simulink model "gm_uz_pmsm_model_6LUT_pd_vnl"  (R2023b)
settings: Solver=FixedStepAuto  StartTime=0.0  StopTime=0.05  RelTol=1e-3
PreLoadFcn:
  | uz_pmsm_model_init_parameter
PostLoadFcn:
  | % Import the data from Excel for a lookup table
  | FluxMapData = readtable('C:\Users\Philipp\ultrazohm\ultrazohm_sw\ip_cores\uz_pmsm_model\FluxMapData_2023-05-26_13-07-57.csv');
  | % Row indices for lookup table
  | d_current_in_d_axis = FluxMapData(8:27,1:end);
  | % Column indices for lookup table
  | q_current_in_d_axis = FluxMapData(29:48,1:end);
  | % Output values for lookup table
  | d_Flux_d_axis = FluxMapData(50:69,1:end);
undefined symbols (not defined in the file or in its folder): ad1, ad2, ad3, ad4, ad5, ad6, aq1, aq2, aq3, aq4, aq5, aq6, d_current_d_Flux, d_current_q_Flux, entkopplung_dynamic, entkopplung_linear, entkopplung_static, Fid1_Giq1, Fid2_Giq2, Flux_d, Flux_q, friction_coefficient, inertia, Ki_Bo_d, Ki_Bo_q, Kp_Bo_d, Kp_Bo_q, L_d, L_q, Ldq, parameter_nachfuerung, polepair, praediktion_entkopplung_nonlinear, psi_pm, q_current_d_Flux, q_current_q_Flux, R_1, simulate_mechanical, simulate_nonlinear_modell, simulate_open_loop, static_friction_torque, tau_sum, ts, ts_regler
libraries: hdlmdlgenlib x19, simulink x2, slpidlib x2
(part 2 of 4)

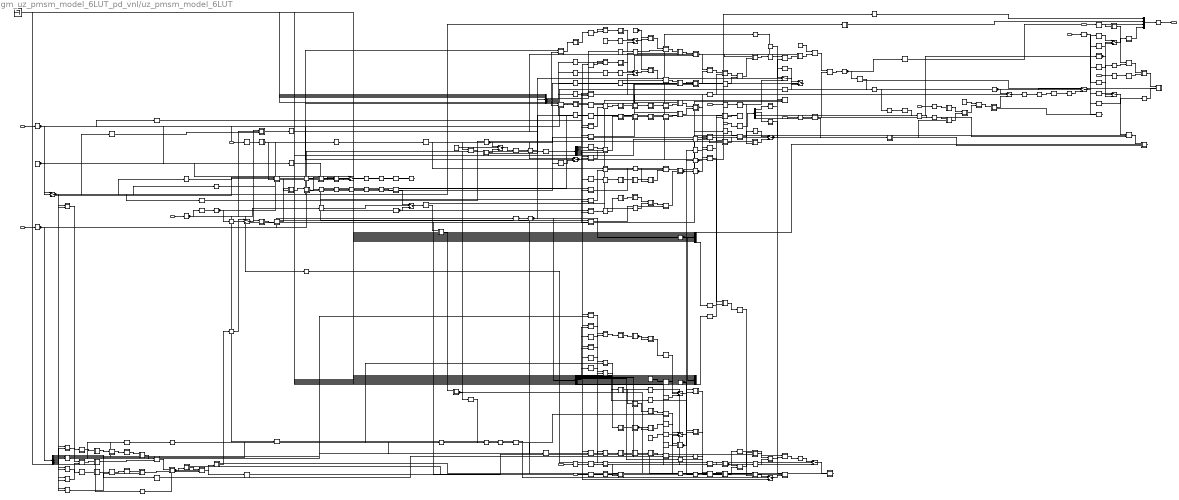
== system gm_uz_pmsm_model_6LUT_pd_vnl/uz_pmsm_model_6LUT ==
  reset_integrators : Inport  OutDataTypeStr=boolean  PortDimensions=1  SampleTime=2e-06
  simulate_mechanical : Inport  Port=2  OutDataTypeStr=boolean  PortDimensions=1  SampleTime=2e-06
  simulate_nonlinear : Inport  Port=3  OutDataTypeStr=boolean  PortDimensions=1  SampleTime=2e-06
  reciprocal_J : Inport  Port=4  OutDataTypeStr=single  PortDimensions=1  SampleTime=2e-06
  mu : Inport  Port=5  OutDataTypeStr=single  PortDimensions=1  SampleTime=2e-06
  M_n0 : Inport  Port=6  OutDataTypeStr=single  PortDimensions=1  SampleTime=2e-06
  R1 : Inport  Port=7  OutDataTypeStr=single  PortDimensions=1  SampleTime=2e-06
  polepairs : Inport  Port=8  OutDataTypeStr=single  PortDimensions=1  SampleTime=2e-06
  Ld : Inport  Port=9  OutDataTypeStr=single  PortDimensions=1  SampleTime=2e-06
  Lq : Inport  Port=10  OutDataTypeStr=single  PortDimensions=1  SampleTime=2e-06
  psi_pm : Inport  Port=11  OutDataTypeStr=single  PortDimensions=1  SampleTime=2e-06
  fitting_parameters : Inport  Port=12  OutDataTypeStr=double  PortDimensions=[14]  SampleTime=2e-06
  inputs : Inport  Port=13  OutDataTypeStr=single  PortDimensions=[4]  SampleTime=2e-06
  Abs : Subsystem
      mask Display: disp('NFP\nabs');
  Constant : Constant  Value=double(0)  OutDataTypeStr=double  SampleTime=1e-08
  Constant1 : Constant  Value=double(1)  OutDataTypeStr=double  SampleTime=1e-08
  Constant11 : Constant  Value=double(1)  OutDataTypeStr=double  SampleTime=1e-08
  Data Type Conversion1 : Subsystem
      mask Display: disp('NFP\nconv');
  Data Type Conversion10 : Subsystem
      mask Display: disp('NFP\nconv');
  Data Type Conversion11 : Subsystem
      mask Display: disp('NFP\nconv');
  Data Type Conversion111 : Subsystem
      mask Display: disp('NFP\nconv');
  Data Type Conversion12 : Subsystem
      mask Display: disp('NFP\nconv');
  Data Type Conversion121 : Subsystem
      mask Display: disp('NFP\nconv');
  Data Type Conversion13 : Subsystem
      mask Display: disp('NFP\nconv');
  Data Type Conversion14 : Subsystem
      mask Display: disp('NFP\nconv');
  Data Type Conversion15 : Subsystem
      mask Display: disp('NFP\nconv');
  Data Type Conversion16 : Subsystem
      mask Display: disp('NFP\nconv');
  Data Type Conversion17 : Subsystem
      mask Display: disp('NFP\nconv');
  Data Type Conversion2 : Subsystem
      mask Display: disp('NFP\nconv');
  Data Type Conversion21 : Subsystem
      mask Display: disp('NFP\nconv');
  Data Type Conversion22 : Subsystem
      mask Display: disp('NFP\nconv');
  Data Type Conversion23 : Subsystem
      mask Display: disp('NFP\nconv');
  Data Type Conversion24 : Subsystem
      mask Display: disp('NFP\nconv');
  Data Type Conversion3 : Subsystem
      mask Display: disp('NFP\nconv');
  Data Type Conversion31 : Subsystem
      mask Display: disp('NFP\nconv');
  Data Type Conversion32 : Subsystem
      mask Display: disp('NFP\nconv');
  Data Type Conversion4 : Subsystem
      mask Display: disp('NFP\nconv');
  Data Type Conversion41 : Subsystem
      mask Display: disp('NFP\nconv');
  Data Type Conversion42 : Subsystem
      mask Display: disp('NFP\nconv');
  Data Type Conversion43 : Subsystem
      mask Display: disp('NFP\nconv');
  Data Type Conversion5 : Subsystem
      mask Display: disp('NFP\nconv');
  Data Type Conversion51 : Subsystem
      mask Display: disp('NFP\nconv');
  Data Type Conversion52 : Subsystem
      mask Display: disp('NFP\nconv');
  Data Type Conversion53 : Subsystem
      mask Display: disp('NFP\nconv');
  Data Type Conversion6 : Subsystem
      mask Display: disp('NFP\nconv');
  Data Type Conversion61 : Subsystem
      mask Display: disp('NFP\nconv');
  Data Type Conversion62 : Subsystem
      mask Display: disp('NFP\nconv');
  Data Type Conversion63 : Subsystem
      mask Display: disp('NFP\nconv');
  Data Type Conversion64 : Subsystem
      mask Display: disp('NFP\nconv');
  Data Type Conversion7 : Subsystem
      mask Display: disp('NFP\nconv');
  Data Type Conversion71 : Subsystem
      mask Display: disp('NFP\nconv');
  Data Type Conversion72 : Subsystem
      mask Display: disp('NFP\nconv');
  Data Type Conversion8 : Subsystem
      mask Display: disp('NFP\nconv');
  Data Type Conversion81 : Subsystem
      mask Display: disp('NFP\nconv');
  Data Type Conversion82 : Subsystem
      mask Display: disp('NFP\nconv');
  Data Type Conversion83 : Subsystem
      mask Display: disp('NFP\nconv');
  Data Type Conversion9 : Subsystem
      mask Display: disp('NFP\nconv');
  Delay : RateTransition  OutPortSampleTimeOpt=Multiple of input port sample time  OutPortSampleTimeMultiple=200
  Delay1_lowered : RateTransition  OutPortSampleTimeOpt=Multiple of input port sample time  OutPortSampleTimeMultiple=200
  Delay1_lowered1 : RateTransition  OutPortSampleTimeOpt=Multiple of input port sample time  OutPortSampleTimeMultiple=200
  Delay1_lowered2 : RateTransition  OutPortSampleTimeOpt=Multiple of input port sample time  OutPortSampleTimeMultiple=200
  Delay1_lowered_absorbed : Delay  DelayLength=0
  Delay1_lowered_absorbed1 : Delay  DelayLength=0
  Delay1_lowered_absorbed2 : Delay  DelayLength=0
  Delay_absorbed : Delay  DelayLength=0
  Divide : Subsystem
      mask Display: disp('NFP\nmul');
  Divide1 : Subsystem
      mask Display: disp('NFP\nmul');
  Divide_recip : Subsystem
      mask Display: disp('NFP\nmath');
  Factor : Subsystem
      mask Display: disp('NFP\nmul');
  Factor_const : Constant  Value=double(1.5)  OutDataTypeStr=double  SampleTime=1e-08
  From1 : hdlmdlgenlib/Buffer
  From1_out1_0_term0 : Terminator
  From1_out1_10_term10 : Terminator
  From1_out1_11_term11 : Terminator
  From1_out1_12_term12 : Terminator
  From1_out1_13_term13 : Terminator
  From1_out1_1_term1 : Terminator
  From1_out1_2_term2 : Terminator
  From1_out1_3_term3 : Terminator
  From1_out1_4_term4 : Terminator
  From1_out1_5_term5 : Terminator
  From1_out1_6_term6 : Terminator
  From1_out1_7_term7 : Terminator
  From1_out1_8_term8 : Terminator
  From1_out1_9_term9 : Terminator
  From2 : hdlmdlgenlib/Buffer
  From2_out1_0_term0 : Terminator
  From2_out1_0_term01 : Terminator
  From2_out1_10_term10 : Terminator
  From2_out1_10_term101 : Terminator
  From2_out1_11_term11 : Terminator
  From2_out1_11_term111 : Terminator
  From2_out1_12_term12 : Terminator
  From2_out1_13_term13 : Terminator
  From2_out1_1_term1 : Terminator
  From2_out1_1_term11 : Terminator
  From2_out1_2_term2 : Terminator
  From2_out1_2_term21 : Terminator
  From2_out1_3_term3 : Terminator
  From2_out1_3_term31 : Terminator
  From2_out1_4_term4 : Terminator
  From2_out1_4_term41 : Terminator
  From2_out1_5_term5 : Terminator
  From2_out1_5_term51 : Terminator
  From2_out1_6_term6 : Terminator
  From2_out1_6_term61 : Terminator
  From2_out1_7_term7 : Terminator
  From2_out1_7_term71 : Terminator
  From2_out1_8_term8 : Terminator
  From2_out1_8_term81 : Terminator
  From2_out1_9_term9 : Terminator
  From2_out1_9_term91 : Terminator
  From3 : hdlmdlgenlib/Buffer
  Gain : Subsystem
      mask Display: disp('NFP\nmul');
  Gain7 : Subsystem
      mask Display: disp('NFP\nmul');
  Gain71 : Subsystem
      mask Display: disp('NFP\nmul');
  Gain7_const : Constant  Value=double(2e-06)  OutDataTypeStr=double  SampleTime=1e-08
  Gain7_const1 : Constant  Value=double(2e-06)  OutDataTypeStr=double  SampleTime=1e-08
  Gain_const : Constant  Value=double(2e-06)  OutDataTypeStr=double  SampleTime=1e-08
  Gain_unaryminus : Subsystem
      mask Display: disp('NFP\numinus');
  Gain_unaryminus1 : Subsystem
      mask Display: disp('NFP\numinus');
  Goto1 : hdlmdlgenlib/Buffer
  Goto2 : hdlmdlgenlib/Buffer
  Initial_Val : Constant  Value=double(0)  OutDataTypeStr=double  SampleTime=1e-08
  Initial_Val1 : Constant  Value=double(0)  OutDataTypeStr=double  SampleTime=1e-08
  Initial_Val2 : Constant  Value=double(0)  OutDataTypeStr=double  SampleTime=1e-08
  Ldd : hdlmdlgenlib/Buffer
  Log : Subsystem
      mask Display: disp('NFP\nmath');
  Log1 : Subsystem
      mask Display: disp('NFP\nmath');
  Log11 : Subsystem
      mask Display: disp('NFP\nmath');
  Log2 : Subsystem
      mask Display: disp('NFP\nmath');
  Lqq : hdlmdlgenlib/Buffer
  M_Mi : hdlmdlgenlib/Buffer
  Product : Subsystem
      mask Display: disp('NFP\nmul');
  Product1 : Subsystem
      mask Display: disp('NFP\nmul');
  Product10 : Subsystem
      mask Display: disp('NFP\nmul');
  Product101 : Subsystem
      mask Display: disp('NFP\nmul');
  Product102 : Subsystem
      mask Display: disp('NFP\nmul');
  Product103 : Subsystem
      mask Display: disp('NFP\nmul');
  Product104 : Subsystem
      mask Display: disp('NFP\nmul');
  Product105 : Subsystem
      mask Display: disp('NFP\nmul');
  Product11 : Subsystem
      mask Display: disp('NFP\nmul');
  Product110 : Subsystem
      mask Display: disp('NFP\nmul');
  Product111 : Subsystem
      mask Display: disp('NFP\nmul');
  Product112 : Subsystem
      mask Display: disp('NFP\nmul');
  Product113 : Subsystem
      mask Display: disp('NFP\nmul');
  Product12 : Subsystem
      mask Display: disp('NFP\nmul');
  Product121 : Subsystem
      mask Display: disp('NFP\nmul');
  Product122 : Subsystem
      mask Display: disp('NFP\nmul');
  Product13 : Subsystem
      mask Display: disp('NFP\nmul');
  Product131 : Subsystem
      mask Display: disp('NFP\nmul');
  Product132 : Subsystem
      mask Display: disp('NFP\nmul');
  Product133 : Subsystem
      mask Display: disp('NFP\nmul');
  Product14 : Subsystem
      mask Display: disp('NFP\nmul');
  Product141 : Subsystem
      mask Display: disp('NFP\nmul');
  Product15 : Subsystem
      mask Display: disp('NFP\nmul');
  Product151 : Subsystem
      mask Display: disp('NFP\nmul');
  Product16 : Subsystem
      mask Display: disp('NFP\nmul');
  Product161 : Subsystem
      mask Display: disp('NFP\nmul');
  Product162 : Subsystem
      mask Display: disp('NFP\nmul');
  Product17 : Subsystem
      mask Display: disp('NFP\nmul');
  Product18 : Subsystem
      mask Display: disp('NFP\nmul');
  Product19 : Subsystem
      mask Display: disp('NFP\nmul');
  Product2 : Subsystem
      mask Display: disp('NFP\nmul');
  Product20 : Subsystem
      mask Display: disp('NFP\nmul');
  Product201 : Subsystem
      mask Display: disp('NFP\nmul');
  Product202 : Subsystem
      mask Display: disp('NFP\nmul');
  Product203 : Subsystem
      mask Display: disp('NFP\nmul');
  Product204 : Subsystem
      mask Display: disp('NFP\nmul');
  Product205 : Subsystem
      mask Display: disp('NFP\nmul');
  Product206 : Subsystem
      mask Display: disp('NFP\nmul');
  Product207 : Subsystem
      mask Display: disp('NFP\nmul');
  Product21 : Subsystem
      mask Display: disp('NFP\nmul');
  Product211 : Subsystem
      mask Display: disp('NFP\nmul');
  Product22 : Subsystem
      mask Display: disp('NFP\nmul');
  Product23 : Subsystem
      mask Display: disp('NFP\nmul');
  Product24 : Subsystem
      mask Display: disp('NFP\nmul');
  Product25 : Subsystem
      mask Display: disp('NFP\nmul');
  Product3 : Subsystem
      mask Display: disp('NFP\nmul');
  Product31 : Subsystem
      mask Display: disp('NFP\nmul');
  Product32 : Subsystem
      mask Display: disp('NFP\nmul');
  Product33 : Subsystem
      mask Display: disp('NFP\nmul');
  Product34 : Subsystem
      mask Display: disp('NFP\nmul');
  Product35 : Subsystem
      mask Display: disp('NFP\nmul');
  Product36 : Subsystem
      mask Display: disp('NFP\nmul');
  Product37 : Subsystem
      mask Display: disp('NFP\nmul');
  Product4 : Subsystem
      mask Display: disp('NFP\nmul');
  Product41 : Subsystem
      mask Display: disp('NFP\nmul');
  Product42 : Subsystem
      mask Display: disp('NFP\nmul');
  Product43 : Subsystem
      mask Display: disp('NFP\nmul');
  Product5 : Subsystem
      mask Display: disp('NFP\nmul');
  Product51 : Subsystem
      mask Display: disp('NFP\nmul');
  Product52 : Subsystem
      mask Display: disp('NFP\nmul');
  Product6 : Subsystem
      mask Display: disp('NFP\nmul');
  Product61 : Subsystem
      mask Display: disp('NFP\nmul');
  Product7 : Subsystem
      mask Display: disp('NFP\nmul');
  Product71 : Subsystem
      mask Display: disp('NFP\nmul');
  Product7_to_gain : Subsystem
      mask Display: disp('NFP\ngain_pow2');
  Product8 : Subsystem
      mask Display: disp('NFP\nmul');
  Product81 : Subsystem
      mask Display: disp('NFP\nmul');
  Product9 : Subsystem
      mask Display: disp('NFP\nmul');
  Product91 : Subsystem
      mask Display: disp('NFP\nmul');
  Product92 : Subsystem
      mask Display: disp('NFP\nmul');
  Product93 : Subsystem
      mask Display: disp('NFP\nmul');
  Product94 : Subsystem
      mask Display: disp('NFP\nmul');
  Sign1 : Subsystem
      mask Display: disp('NFP\nsignum');
  Sum : Subsystem
      mask Display: disp('NFP\nadd');
  Sum1 : Subsystem
      mask Display: disp('NFP\nadd');
  Sum10 : Subsystem
      mask Display: disp('NFP\nadd');
  Sum101 : Subsystem
      mask Display: disp('NFP\nadd');
  Sum11 : Subsystem
      mask Display: disp('NFP\nadd');
  Sum12 : Subsystem
      mask Display: disp('NFP\nadd');
  Sum13 : Subsystem
      mask Display: disp('NFP\nadd');
  Sum14 : Subsystem
      mask Display: disp('NFP\nadd');
  Sum2 : Subsystem
      mask Display: disp('NFP\nadd');
  Sum21 : Subsystem
      mask Display: disp('NFP\nadd');
  Sum22 : Subsystem
      mask Display: disp('NFP\nadd');
  Sum23 : Subsystem
      mask Display: disp('NFP\nadd');
  Sum24 : Subsystem
      mask Display: disp('NFP\nadd');
  Sum3 : Subsystem
      mask Display: disp('NFP\nadd');
  Sum31 : Subsystem
      mask Display: disp('NFP\nadd');
  Sum32 : Subsystem
      mask Display: disp('NFP\nadd');
  Sum3_stage2 : Subsystem
      mask Display: disp('NFP\nadd');
  Sum3_stage21 : Subsystem
      mask Display: disp('NFP\nadd');
  Sum3_stage3 : Subsystem
      mask Display: disp('NFP\nadd');
  Sum3_stage31 : Subsystem
      mask Display: disp('NFP\nadd');
  Sum3_stage4 : Subsystem
      mask Display: disp('NFP\nadd');
  Sum4 : Subsystem
      mask Display: disp('NFP\nadd');
  Sum41 : Subsystem
      mask Display: disp('NFP\nadd');
  Sum42 : Subsystem
      mask Display: disp('NFP\nadd');
  Sum4_stage2 : Subsystem
      mask Display: disp('NFP\nadd');
  Sum4_stage3 : Subsystem
      mask Display: disp('NFP\nadd');
  Sum4_stage4 : Subsystem
      mask Display: disp('NFP\nadd');
  Sum5 : Subsystem
      mask Display: disp('NFP\nadd');
  Sum51 : Subsystem
      mask Display: disp('NFP\nadd');
  Sum52 : Subsystem
      mask Display: disp('NFP\nadd');
  Sum53 : Subsystem
      mask Display: disp('NFP\nadd');
  Sum6 : Subsystem
      mask Display: disp('NFP\nadd');
  Sum7 : Subsystem
      mask Display: disp('NFP\nadd');
  Sum71 : Subsystem
      mask Display: disp('NFP\nadd');
  Sum8 : Subsystem
      mask Display: disp('NFP\nadd');
  Sum9 : Subsystem
      mask Display: disp('NFP\nadd');
  Switch{,1..6,11} (8 alike) : Switch  Criteria=u2 ~= 0  Threshold=double(0)  OutDataTypeStr=double  SampleTime=1e-08  SaturateOnIntegerOverflow=off  InputSameDT=off
  Tanh : Subsystem
      mask Display: disp('NFP\ntrig');
  Tanh1 : Subsystem
      mask Display: disp('NFP\ntrig');
  Tanh11 : Subsystem
      mask Display: disp('NFP\ntrig');
  Tanh12 : Subsystem
      mask Display: disp('NFP\ntrig');
  Tanh13 : Subsystem
      mask Display: disp('NFP\ntrig');
  Tanh2 : Subsystem
      mask Display: disp('NFP\ntrig');
  Tanh21 : Subsystem
      mask Display: disp('NFP\ntrig');
  Tanh3 : Subsystem
      mask Display: disp('NFP\ntrig');
  Tanh31 : Subsystem
      mask Display: disp('NFP\ntrig');
  Tanh4 : Subsystem
      mask Display: disp('NFP\ntrig');
  Tanh41 : Subsystem
      mask Display: disp('NFP\ntrig');
  Tanh5 : Subsystem
      mask Display: disp('NFP\ntrig');
  Unit Delay : RateTransition  OutPortSampleTimeOpt=Multiple of input port sample time  OutPortSampleTimeMultiple=200
  Unit Delay1 : RateTransition  OutPortSampleTimeOpt=Multiple of input port sample time  OutPortSampleTimeMultiple=200
  Unit Delay1_absorbed : Delay  DelayLength=0
  Unit Delay_absorbed : Delay  DelayLength=0
  crp_out_delay{,1..5} (6 alike) : Delay  DelayLength=double(1)  InitialCondition=0  SampleTime=1e-08
  default_value{,1..4} (5 alike) : Constant  Value=double(1)  OutDataTypeStr=double  SampleTime=1e-08
  delayMatch{,1..16,18..20,22..41,43..45,47..51,53..57} (53 alike) : Delay  DelayLength=double(1)  InitialCondition=0  SampleTime=1e-08
  delayMatch17 : Delay  DelayLength=double(41)  InitialCondition=0  SampleTime=1e-08
  delayMatch21 : Delay  DelayLength=double(41)  InitialCondition=0  SampleTime=1e-08
  delayMatch42 : Delay  DelayLength=double(35)  InitialCondition=0  SampleTime=1e-08
  delayMatch46 : Delay  DelayLength=double(35)  InitialCondition=0  SampleTime=1e-08
  delayMatch52 : Delay  DelayLength=double(108)  InitialCondition=0  SampleTime=1e-08
  fitting_parameters_12_term12 : Terminator
  fitting_parameters_13_term13 : Terminator
  in0_repeat : RateTransition  Integrity=off  Deterministic=off  OutPortSampleTimeOpt=Multiple of input port sample time  OutPortSampleTimeMultiple=1/200
  in10_repeat : RateTransition  Integrity=off  Deterministic=off  OutPortSampleTimeOpt=Multiple of input port sample time  OutPortSampleTimeMultiple=1/200
  in11_repeat : RateTransition  Integrity=off  Deterministic=off  OutPortSampleTimeOpt=Multiple of input port sample time  OutPortSampleTimeMultiple=1/200
  in12_repeat : RateTransition  Integrity=off  Deterministic=off  OutPortSampleTimeOpt=Multiple of input port sample time  OutPortSampleTimeMultiple=1/200
  in13_repeat : RateTransition  Integrity=off  Deterministic=off  OutPortSampleTimeOpt=Multiple of input port sample time  OutPortSampleTimeMultiple=1/200
  in14_repeat : RateTransition  Integrity=off  Deterministic=off  OutPortSampleTimeOpt=Multiple of input port sample time  OutPortSampleTimeMultiple=1/200
  in15_repeat : RateTransition  Integrity=off  Deterministic=off  OutPortSampleTimeOpt=Multiple of input port sample time  OutPortSampleTimeMultiple=1/200
  in16_repeat : RateTransition  Integrity=off  Deterministic=off  OutPortSampleTimeOpt=Multiple of input port sample time  OutPortSampleTimeMultiple=1/200
  in17_repeat : RateTransition  Integrity=off  Deterministic=off  OutPortSampleTimeOpt=Multiple of input port sample time  OutPortSampleTimeMultiple=1/200
  in18_repeat : RateTransition  Integrity=off  Deterministic=off  OutPortSampleTimeOpt=Multiple of input port sample time  OutPortSampleTimeMultiple=1/200
  in1_repeat : RateTransition  Integrity=off  Deterministic=off  OutPortSampleTimeOpt=Multiple of input port sample time  OutPortSampleTimeMultiple=1/200
  in2_repeat : RateTransition  Integrity=off  Deterministic=off  OutPortSampleTimeOpt=Multiple of input port sample time  OutPortSampleTimeMultiple=1/200
  in3_repeat : RateTransition  Integrity=off  Deterministic=off  OutPortSampleTimeOpt=Multiple of input port sample time  OutPortSampleTimeMultiple=1/200
  in4_repeat : RateTransition  Integrity=off  Deterministic=off  OutPortSampleTimeOpt=Multiple of input port sample time  OutPortSampleTimeMultiple=1/200
  in5_repeat : RateTransition  Integrity=off  Deterministic=off  OutPortSampleTimeOpt=Multiple of input port sample time  OutPortSampleTimeMultiple=1/200
  in6_repeat : RateTransition  Integrity=off  Deterministic=off  OutPortSampleTimeOpt=Multiple of input port sample time  OutPortSampleTimeMultiple=1/200
  in7_repeat : RateTransition  Integrity=off  Deterministic=off  OutPortSampleTimeOpt=Multiple of input port sample time  OutPortSampleTimeMultiple=1/200
  in8_repeat : RateTransition  Integrity=off  Deterministic=off  OutPortSampleTimeOpt=Multiple of input port sample time  OutPortSampleTimeMultiple=1/200
  in9_repeat : RateTransition  Integrity=off  Deterministic=off  OutPortSampleTimeOpt=Multiple of input port sample time  OutPortSampleTimeMultiple=1/200
  mux : Mux
  psi_d_approx : hdlmdlgenlib/Buffer
  psi_q_approx : hdlmdlgenlib/Buffer
  reset_in : Switch  Criteria=u2 ~= 0  Threshold=double(0)  OutDataTypeStr=double  SampleTime=1e-08  SaturateOnIntegerOverflow=off  InputSameDT=off
  reset_in1 : Switch  Criteria=u2 ~= 0  Threshold=double(0)  OutDataTypeStr=double  SampleTime=1e-08  SaturateOnIntegerOverflow=off  InputSameDT=off
  reset_in2 : Switch  Criteria=u2 ~= 0  Threshold=double(0)  OutDataTypeStr=double  SampleTime=1e-08  SaturateOnIntegerOverflow=off  InputSameDT=off
  reset_out : Switch  Criteria=u2 ~= 0  Threshold=double(0)  OutDataTypeStr=double  SampleTime=1e-08  SaturateOnIntegerOverflow=off  InputSameDT=off
  reset_out1 : Switch  Criteria=u2 ~= 0  Threshold=double(0)  OutDataTypeStr=double  SampleTime=1e-08  SaturateOnIntegerOverflow=off  InputSameDT=off
  reset_out2 : Switch  Criteria=u2 ~= 0  Threshold=double(0)  OutDataTypeStr=double  SampleTime=1e-08  SaturateOnIntegerOverflow=off  InputSameDT=off
  select_signal{,1..4} (5 alike) : Constant  Value=double(1)  OutDataTypeStr=boolean  SampleTime=1e-08
  t : RateTransition  OutPortSampleTimeOpt=Multiple of input port sample time  OutPortSampleTimeMultiple=200
  t{1..6} (6 alike) : Demux  Outputs=14
  t{8..16} (9 alike) : hdlmdlgenlib/Buffer
  t7 : Demux
  zero_protection{,1..4} (5 alike) : Switch  Criteria=u2 ~= 0  Threshold=double(0)  OutDataTypeStr=double  SampleTime=1e-08  SaturateOnIntegerOverflow=off  InputSameDT=off
  outputs : Outport  SampleTime=2e-06
  wires:
  default_value4/1 -> zero_protection4/3
  zero_protection4/1 -> Divide1/2(In2)
  default_value3/1 -> zero_protection3/3
  zero_protection3/1 -> Product162/2(In2)
  default_value2/1 -> zero_protection2/3
  zero_protection2/1 -> Product133/2(In2)
  default_value1/1 -> zero_protection1/3
  zero_protection1/1 -> Product132/2(In2)
  default_value/1 -> zero_protection/3
  zero_protection/1 -> Product161/2(In2)
  reset_out1/1 -> delayMatch9/1, delayMatch34/1, Sign1/1(In1), Abs/1(In1), delayMatch56/1
  delayMatch57/1 -> reset_in1/2
  reset_out/1 -> Data Type Conversion15/1(In1), delayMatch32/1, Product8/1(In1), Product8/2(In2), Product5/1(In1), Product4/1(In1), Product10/1(In1), Product24/1(In1), Product11/1(In1), Product51/1(In1), Product61/1(In1), Product25/1(In1), delayMatch14/1, delayMatch41/1, delayMatch53/1
  select_signal4/1 -> delayMatch52/1
  select_signal3/1 -> delayMatch46/1
  select_signal2/1 -> delayMatch42/1
  delayMatch51/1 -> Switch11/2
  From3/1 -> delayMatch15/1, delayMatch31/1
  delayMatch54/1 -> reset_in/2
  reset_out2/1 -> Data Type Conversion111/1(In1), delayMatch33/1, Sum/1(In1), Sum1/1(In1), Sum11/1(In1), Sum2/1(In1), Sum3/1(In1), Sum6/1(In1), delayMatch/1, delayMatch30/1, delayMatch27/1
  delayMatch40/1 -> Switch4/2
  delayMatch26/1 -> Switch2/2
  select_signal/1 -> delayMatch21/1
  delayMatch23/1 -> Product32/2(In2)
  select_signal1/1 -> delayMatch17/1
  delayMatch19/1 -> Product19/2(In2)
  delayMatch31/1 -> Switch5/2
  delayMatch41/1 -> Product92/1(In1)
  delayMatch35/1 -> Switch1/2
  delayMatch34/1 -> Switch1/1
  delayMatch30/1 -> Product52/1(In1)
  delayMatch52/1 -> zero_protection4/2
  delayMatch46/1 -> zero_protection3/2
  delayMatch42/1 -> zero_protection2/2
  delayMatch17/1 -> zero_protection1/2
  delayMatch21/1 -> zero_protection/2
  Gain/1(Out1) -> Sum31/1(In1)
  Product7_to_gain/1(Out1) -> Sum3_stage2/2(In2)
  Data Type Conversion14/1(Out1) -> Product93/2(In2), Product131/2(In2)
  Product131/1(Out1) -> Product37/1(In1), Product21/2(In2)
  Sum3_stage4/1(Out1) -> Divide/1(In1)
  Sum3_stage31/1(Out1) -> Sum3_stage4/1(In1)
  Sum3_stage21/1(Out1) -> Sum3_stage31/1(In1)
  Divide_recip/1(Out1) -> Divide/2(In2)
  Sum53/1(Out1) -> reset_in2/3
  Data Type Conversion111/1(Out1) -> mux/1
  Product36/1(Out1) -> Sum32/1(In1)
  Sum32/1(Out1) -> Factor/2(In2)
  Sum9/1(Out1) -> crp_out_delay2/1
  Product43/1(Out1) -> Sum9/2(In2)
  Sum52/1(Out1) -> Product43/1(In1)
  Data Type Conversion64/1(Out1) -> Sum52/2(In2)
  Product122/1(Out1) -> Sum52/1(In1)
  Abs/1(Out1) -> delayMatch36/1
  Sign1/1(Out1) -> delayMatch37/1
  Data Type Conversion121/1(Out1) -> Switch1/3, Switch/3
  Data Type Conversion13/1(Out1) -> Sum14/2(In2)
  Sum14/1(Out1) -> Product112/2(In2)
  Product112/1(Out1) -> Gain/2(In2)
  Data Type Conversion72/1(Out1) -> Product112/1(In1)
  Sum31/1(Out1) -> reset_in1/3
  Data Type Conversion10/1(Out1) -> Sum4_stage2/1(In1)
  Sum4_stage4/1(Out1) -> Divide1/1(In1)
  Sum4_stage3/1(Out1) -> Sum4_stage4/1(In1)
  Sum4_stage2/1(Out1) -> Sum4_stage3/1(In1)
  Sum51/1(Out1) -> reset_in/3
  Product92/1(Out1) -> Sum4_stage4/2(In2)
  Data Type Conversion9/1(Out1) -> Product42/1(In1), Product92/2(In2)
  Product42/1(Out1) -> Sum3_stage21/2(In2)
  Product110/1(Out1) -> Switch6/3
  Sum42/1(Out1) -> Sum24/1(In1), t16/1
  Sum24/1(Out1) -> t11/1, t15/1
  Product206/1(Out1) -> Product207/1(In1)
  Product121/1(Out1) -> Switch3/1
  Product111/1(Out1) -> Switch4/1
  Product204/1(Out1) -> Product205/1(In1)
  Sum23/1(Out1) -> t10/1, t14/1
  Product104/1(Out1) -> Product105/1(In1)
  Sum8/1(Out1) -> Switch5/3
  Data Type Conversion43/1(Out1) -> Sum8/2(In2)
  Product52/1(Out1) -> Sum8/1(In1)
  Data Type Conversion24/1(Out1) -> Switch2/3, Product52/2(In2)
  Product19/1(Out1) -> Sum22/1(In1), t13/1
  Product18/1(Out1) -> Product19/1(In1)
  Product102/1(Out1) -> Product103/1(In1)
  Product16/1(Out1) -> Product17/1(In1)
  Sum13/1(Out1) -> Sum10/1(In1), Sum21/1(In1)
  Product202/1(Out1) -> Product203/1(In1)
  Product20/1(Out1) -> Product201/1(In1)
  Data Type Conversion23/1(Out1) -> Product35/1(In1)
  Tanh13/1(Out1) -> Data Type Conversion23/1(In1)
  Data Type Conversion71/1(Out1) -> Tanh13/1(In1)
  Product25/1(Out1) -> Data Type Conversion71/1(In1)
  Sum12/1(Out1) -> Sum24/2(In2)
  Product61/1(Out1) -> Sum12/2(In2)
  Product51/1(Out1) -> Sum42/1(In1)
  Product13/1(Out1) -> Sum42/2(In2)
  Data Type Conversion32/1(Out1) -> Product13/1(In1)
  Tanh5/1(Out1) -> Data Type Conversion32/1(In1)
  Data Type Conversion83/1(Out1) -> Tanh5/1(In1)
  Product11/1(Out1) -> Data Type Conversion83/1(In1)
  Product81/1(Out1) -> Product91/1(In1)
  Product91/1(Out1) -> Sum5/2(In2)
  Data Type Conversion42/1(Out1) -> Product91/2(In2)
  Log11/1(Out1) -> Data Type Conversion42/1(In1)
  Tanh21/1(Out1) -> Log11/1(In1)
  Data Type Conversion63/1(Out1) -> Tanh21/1(In1)
  Product211/1(Out1) -> Product41/1(In1)
  Product41/1(Out1) -> Sum5/1(In1)
  Data Type Conversion12/1(Out1) -> Product41/2(In2)
  Log2/1(Out1) -> Data Type Conversion12/1(In1)
  Tanh41/1(Out1) -> Log2/1(In1)
  Data Type Conversion53/1(Out1) -> Tanh41/1(In1)
  Sum21/1(Out1) -> Product202/1(In1)
  Sum41/1(Out1) -> Sum21/2(In2)
  Product33/1(Out1) -> Product34/1(In1)
  Product162/1(Out1) -> Product33/1(In1)
  Data Type Conversion22/1(Out1) -> zero_protection3/1
  Product151/1(Out1) -> Data Type Conversion22/1(In1)
  Tanh12/1(Out1) -> Product151/1(In1), Product151/2(In2)
  Data Type Conversion41/1(Out1) -> Tanh12/1(In1)
  Product24/1(Out1) -> Data Type Conversion41/1(In1)
  Product133/1(Out1) -> Product16/1(In1)
  Data Type Conversion62/1(Out1) -> zero_protection2/1
  Product141/1(Out1) -> Data Type Conversion62/1(In1)
  Tanh31/1(Out1) -> Product141/1(In1), Product141/2(In2)
  Data Type Conversion52/1(Out1) -> Tanh31/1(In1)
  Product10/1(Out1) -> Data Type Conversion52/1(In1)
  Data Type Conversion31/1(Out1) -> Switch11/3, Product110/2(In2)
  Product9/1(Out1) -> Data Type Conversion61/1(In1)
  Sum2/1(Out1) -> Product9/1(In1)
  Data Type Conversion61/1(Out1) -> Tanh4/1(In1)
  Tanh4/1(Out1) -> Product14/1(In1), Product14/2(In2)
  Product14/1(Out1) -> Data Type Conversion21/1(In1)
  Data Type Conversion21/1(Out1) -> zero_protection1/1
  Product132/1(Out1) -> Product18/1(In1)
  Product161/1(Out1) -> Product31/1(In1)
  Data Type Conversion11/1(Out1) -> zero_protection/1
  Product15/1(Out1) -> Data Type Conversion11/1(In1)
  Tanh11/1(Out1) -> Product15/1(In1), Product15/2(In2)
  Data Type Conversion82/1(Out1) -> Tanh11/1(In1)
  Product23/1(Out1) -> Data Type Conversion82/1(In1)
  Sum11/1(Out1) -> Product23/1(In1)
  Product31/1(Out1) -> Product32/1(In1)
  Sum3_stage2/1(Out1) -> Sum3_stage3/1(In1)
  Product6/1(Out1) -> Sum3_stage2/1(In1)
  Data Type Conversion4/1(Out1) -> Product6/1(In1)
  Log/1(Out1) -> Data Type Conversion4/1(In1)
  Tanh2/1(Out1) -> Log/1(In1)
  Data Type Conversion7/1(Out1) -> Tanh2/1(In1)
  Product4/1(Out1) -> Data Type Conversion7/1(In1)
  Product113/1(Out1) -> Product12/2(In2)
  Product12/1(Out1) -> Sum3_stage3/2(In2)
  Data Type Conversion1/1(Out1) -> Product12/1(In1)
  Log1/1(Out1) -> Data Type Conversion1/1(In1)
  Tanh3/1(Out1) -> Log1/1(In1)
  Data Type Conversion81/1(Out1) -> Tanh3/1(In1)
  Product5/1(Out1) -> Data Type Conversion81/1(In1)
  Product7/1(Out1) -> Product7_to_gain/1(In1)
  Product8/1(Out1) -> Product7/1(In1)
  Product94/1(Out1) -> Product6/2(In2)
  Data Type Conversion3/1(Out1) -> Product3/1(In1)
  Tanh1/1(Out1) -> Data Type Conversion3/1(In1)
  Data Type Conversion6/1(Out1) -> Tanh1/1(In1)
  Product22/1(Out1) -> Data Type Conversion6/1(In1)
  Sum1/1(Out1) -> Product22/1(In1)
  Product1/1(Out1) -> Sum23/1(In1), t12/1
  Data Type Conversion2/1(Out1) -> Product1/1(In1)
  Tanh/1(Out1) -> Data Type Conversion2/1(In1)
  Data Type Conversion51/1(Out1) -> Tanh/1(In1)
  Product/1(Out1) -> Data Type Conversion51/1(In1)
  Sum/1(Out1) -> Product/1(In1)
  Product2/1(Out1) -> Sum32/2(In2)
  Data Type Conversion8/1(Out1) -> Sum3_stage21/1(In1)
  Data Type Conversion5/1(Out1) -> Product122/1(In1)
  Gain7_const1/1 -> Gain71/1(In1)
  Factor_const/1 -> Factor/1(In1)
  Gain_const/1 -> Gain/1(In1)
  Gain7_const/1 -> Gain7/1(In1)
  t6/14 -> From1_out1_13_term13/1
  t6/13 -> delayMatch24/1
  t6/12 -> From1_out1_11_term11/1
  t6/11 -> From1_out1_10_term10/1
  t6/10 -> From1_out1_9_term9/1
  t6/9 -> From1_out1_8_term8/1
  t6/8 -> From1_out1_7_term7/1
  t6/7 -> From1_out1_6_term6/1
  t6/5 -> delayMatch20/1, delayMatch23/1
  t6/4 -> delayMatch22/1
  t6/2 -> delayMatch16/1, delayMatch19/1
  t6/1 -> delayMatch18/1
  t5/14 -> delayMatch38/1
  t5/13 -> From2_out1_12_term12/1
  t5/12 -> From2_out1_11_term111/1
  t5/11 -> From2_out1_10_term101/1
  t5/10 -> From2_out1_9_term91/1
  t5/9 -> From2_out1_8_term81/1
  t5/8 -> From2_out1_7_term71/1
  t5/7 -> From2_out1_6_term61/1
  t5/6 -> From2_out1_5_term51/1
  t5/5 -> From2_out1_4_term41/1
  t5/4 -> From2_out1_3_term3/1
  t5/3 -> From2_out1_2_term2/1
  t5/2 -> From2_out1_1_term1/1
  t5/1 -> From2_out1_0_term01/1
  t4/14 -> From2_out1_13_term13/1
  t4/13 -> delayMatch7/1
  t4/12 -> From2_out1_11_term11/1
  t4/11 -> From2_out1_10_term10/1
  t4/10 -> From2_out1_9_term9/1
  t4/9 -> From2_out1_8_term8/1
  t4/8 -> From2_out1_7_term7/1
  t4/7 -> From2_out1_6_term6/1
  t4/6 -> From2_out1_5_term5/1
  t4/5 -> From2_out1_4_term4/1
  t4/4 -> From2_out1_3_term31/1
  t4/3 -> From2_out1_2_term21/1
  t4/2 -> From2_out1_1_term11/1
  t4/1 -> From2_out1_0_term0/1
  t3/14 -> delayMatch50/1
  t3/13 -> From1_out1_12_term12/1
  t3/12 -> delayMatch49/1
  t3/11 -> Product24/2(In2), delayMatch48/1
  t3/10 -> delayMatch47/1
  t3/9 -> delayMatch45/1
  t3/8 -> Product10/2(In2), delayMatch44/1
  t3/7 -> delayMatch43/1
  t3/6 -> From1_out1_5_term5/1
  t3/5 -> From1_out1_4_term4/1
  t3/4 -> From1_out1_3_term3/1
  t3/3 -> From1_out1_2_term2/1
  t3/2 -> From1_out1_1_term1/1
  t3/1 -> From1_out1_0_term0/1
  t2/14 -> delayMatch13/1
  t2/13 -> fitting_parameters_12_term12/1
  t2/10 -> delayMatch6/1
  t2/7 -> delayMatch5/1
  t2/5 -> Product81/2(In2), delayMatch12/1
  t2/2 -> Product211/2(In2), delayMatch11/1
  t1/14 -> fitting_parameters_13_term13/1
  t1/13 -> delayMatch29/1
  t1/5 -> delayMatch3/1
  t1/4 -> delayMatch4/1
  t1/2 -> delayMatch1/1
  t1/1 -> delayMatch2/1
  delayMatch55/1 -> Sum14/1(In1)
  delayMatch28/1 -> reset_in2/2
  delayMatch8/1 -> Product121/2(In2)
  delayMatch39/1 -> Product111/1(In1)
  delayMatch25/1 -> Switch3/2
  delayMatch10/1 -> Switch/2
  Product37/1(Out1) -> Sum3_stage4/2(In2)
  Divide/1(Out1) -> crp_out_delay/1, Gain71/2(In2)
  Gain71/1(Out1) -> Sum53/1(In1)
  reset_in2/1 -> crp_out_delay1/1
  Initial_Val2/1 -> reset_in2/1, reset_out2/1
  delayMatch27/1 -> Sum53/2(In2)
  delayMatch/1 -> Product42/2(In2)
  delayMatch33/1 -> Product2/1(In1)
  Data Type Conversion15/1(Out1) -> mux/2
  delayMatch32/1 -> Product36/2(In2)
  Factor/1(Out1) -> Product93/1(In1)
  Product93/1(Out1) -> M_Mi/1
  M_Mi/1 -> Data Type Conversion16/1(In1), Sum9/1(In1)
  delayMatch36/1 -> Product122/2(In2)
  delayMatch37/1 -> Product43/2(In2)
  delayMatch9/1 -> Switch/1
  Switch/1 -> Product131/1(In1)
  t7/4 -> Data Type Conversion13/1(In1)
  t7/3 -> Data Type Conversion121/1(In1)
  t7/2 -> Data Type Conversion10/1(In1)
  t7/1 -> Data Type Conversion8/1(In1)
  reset_in1/1 -> crp_out_delay5/1
  Initial_Val1/1 -> reset_in1/1, reset_out1/1
  delayMatch56/1 -> Sum31/2(In2)
  Divide1/1(Out1) -> crp_out_delay3/1, Gain7/2(In2)
  Gain7/1(Out1) -> Sum51/1(In1)
  reset_in/1 -> crp_out_delay4/1
  Initial_Val/1 -> reset_in/1, reset_out/1
  delayMatch53/1 -> Sum51/2(In2)
  delayMatch14/1 -> Product110/1(In1)
  Switch6/1 -> Product2/2(In2), Product37/2(In2)
  psi_q_approx/1 -> Switch6/1
  Sum101/1(Out1) -> psi_q_approx/1
  t16/1 -> Sum101/1(In1)
  t15/1 -> Product20/1(In1)
  t11/1 -> Product204/2(In2), Product206/2(In2)
  Product207/1(Out1) -> Gain_unaryminus1/1(In1)
  Gain_unaryminus1/1(Out1) -> Product121/1(In1)
  Switch3/1 -> Sum3_stage31/2(In2)
  Constant/1 -> Switch4/3, Switch3/3
  Switch4/1 -> Sum4_stage2/2(In2)
  Gain_unaryminus/1(Out1) -> Product111/2(In2)
  Product205/1(Out1) -> Gain_unaryminus/1(In1)
  t10/1 -> Product204/1(In1), Product206/1(In1)
  t14/1 -> Product104/1(In1)
  Product105/1(Out1) -> Sum71/2(In2)
  Sum71/1(Out1) -> psi_d_approx/1
  psi_d_approx/1 -> Switch5/1
  Switch5/1 -> Product36/1(In1), Product21/1(In1)
  Switch2/1 -> Divide_recip/1(In1)
  Ldd/1 -> Switch2/1
  Sum7/1(Out1) -> Ldd/1
  t13/1 -> Sum7/1(In1)
  Sum22/1(Out1) -> Product102/1(In1)
  Product103/1(Out1) -> Sum7/2(In2)
  delayMatch24/1 -> Product103/2(In2)
  t6/6 -> Sum11/2(In2)
  delayMatch20/1 -> Product23/2(In2)
  delayMatch22/1 -> Product31/2(In2)
  t6/3 -> Sum2/2(In2)
  delayMatch16/1 -> Product9/2(In2)
  delayMatch18/1 -> Product18/2(In2)
  From1/1 -> t3/1, t6/1
  Goto1/1 -> From1/1, From2/1
  From2/1 -> t4/1, t5/1
  delayMatch38/1 -> Product205/2(In2)
  delayMatch7/1 -> Product207/2(In2)
  delayMatch50/1 -> Product203/2(In2)
  delayMatch49/1 -> Sum41/2(In2)
  delayMatch48/1 -> Product34/2(In2)
  delayMatch47/1 -> Product33/2(In2)
  delayMatch45/1 -> Sum13/2(In2)
  delayMatch44/1 -> Product17/2(In2)
  delayMatch43/1 -> Product16/2(In2)
  Product17/1(Out1) -> Sum13/1(In1)
  Sum10/1(Out1) -> Lqq/1
  Product203/1(Out1) -> Sum10/2(In2)
  t8/1 -> Product202/2(In2)
  Sum5/1(Out1) -> Product20/2(In2), t8/1
  Product201/1(Out1) -> Sum101/2(In2)
  delayMatch13/1 -> Product201/2(In2)
  t2/12 -> Product61/2(In2)
  t2/11 -> Product25/2(In2)
  delayMatch6/1 -> Product35/2(In2)
  t2/9 -> Product51/2(In2)
  t2/8 -> Product11/2(In2)
  delayMatch5/1 -> Product13/2(In2)
  t2/6 -> Sum6/2(In2)
  delayMatch12/1 -> Product101/1(In1)
  t2/4 -> Product81/1(In1)
  t2/3 -> Sum3/2(In2)
  delayMatch11/1 -> Product71/1(In1)
  t2/1 -> Product211/1(In1)
  Product35/1(Out1) -> Sum12/1(In1)
  Product101/1(Out1) -> Data Type Conversion63/1(In1)
  Sum6/1(Out1) -> Product101/2(In2)
  Product71/1(Out1) -> Data Type Conversion53/1(In1)
  Sum3/1(Out1) -> Product71/2(In2)
  Product34/1(Out1) -> Sum41/1(In1)
  Constant11/1 -> Product162/1(In1), Product133/1(In1)
  Lqq/1 -> Switch11/1
  Switch11/1 -> zero_protection4/1
  Constant1/1 -> Product132/1(In1), Product161/1(In1)
  Product32/1(Out1) -> Sum22/2(In2)
  t9/1 -> Product102/2(In2)
  Sum3_stage3/1(Out1) -> Product104/2(In2), t9/1
  delayMatch29/1 -> Product105/2(In2)
  t1/12 -> Sum4/2(In2)
  t1/11 -> Product113/2(In2), Product5/2(In2)
  t1/10 -> Product113/1(In1)
  t1/9 -> Sum4/1(In1)
  t1/8 -> Product94/2(In2), Product4/2(In2)
  t1/7 -> Product94/1(In1)
  t1/6 -> Sum1/2(In2)
  delayMatch3/1 -> Product22/2(In2)
  delayMatch4/1 -> Product3/2(In2)
  t1/3 -> Sum/2(In2)
  delayMatch1/1 -> Product/2(In2)
  delayMatch2/1 -> Product1/2(In2)
  Sum4/1(Out1) -> Product7/2(In2)
  Product3/1(Out1) -> Sum23/2(In2)
  t12/1 -> Sum71/1(In1)
  delayMatch15/1 -> Switch6/2
  Goto2/1 -> From3/1
  Product21/1(Out1) -> Sum4_stage3/2(In2)
  Switch1/1 -> Data Type Conversion17/1(In1)
  Data Type Conversion17/1(Out1) -> mux/4
  Data Type Conversion16/1(Out1) -> mux/3
  crp_out_delay5/1 -> Delay1_lowered1/1
  crp_out_delay4/1 -> Delay1_lowered2/1
  crp_out_delay3/1 -> Unit Delay1/1
  crp_out_delay2/1 -> Delay/1
  crp_out_delay1/1 -> Delay1_lowered/1
  crp_out_delay/1 -> Unit Delay/1
  in3_repeat/1 -> delayMatch39/1
  Unit Delay_absorbed/1 -> in3_repeat/1
  Unit Delay/1 -> Unit Delay_absorbed/1
  in8_repeat/1 -> delayMatch8/1
  Unit Delay1_absorbed/1 -> in8_repeat/1
  Unit Delay1/1 -> Unit Delay1_absorbed/1
  in11_repeat/1 -> reset_out/3
  Delay1_lowered_absorbed2/1 -> in11_repeat/1
  Delay1_lowered2/1 -> Delay1_lowered_absorbed2/1
  in12_repeat/1 -> reset_out1/3
  Delay1_lowered_absorbed1/1 -> in12_repeat/1
  Delay1_lowered1/1 -> Delay1_lowered_absorbed1/1
  in14_repeat/1 -> delayMatch55/1
  Delay_absorbed/1 -> in14_repeat/1
  Delay/1 -> Delay_absorbed/1
  in17_repeat/1 -> reset_out2/3
  Delay1_lowered_absorbed/1 -> in17_repeat/1
  Delay1_lowered/1 -> Delay1_lowered_absorbed/1
  mux/1 -> t/1
  in18_repeat/1 -> Data Type Conversion14/1(In1)
  in16_repeat/1 -> Data Type Conversion64/1(In1)
  in15_repeat/1 -> t7/1
  in13_repeat/1 -> Data Type Conversion72/1(In1)
  in10_repeat/1 -> reset_out/2, reset_out2/2, reset_out1/2, delayMatch28/1, delayMatch54/1, delayMatch57/1
  in9_repeat/1 -> Data Type Conversion9/1(In1)
  in7_repeat/1 -> Data Type Conversion43/1(In1)
  in6_repeat/1 -> Data Type Conversion24/1(In1)
  in5_repeat/1 -> Data Type Conversion31/1(In1)
  in4_repeat/1 -> Goto1/1, t1/1, t2/1
  in2_repeat/1 -> Goto2/1, delayMatch25/1, delayMatch26/1, delayMatch40/1, delayMatch51/1
  in1_repeat/1 -> delayMatch10/1, delayMatch35/1
  in0_repeat/1 -> Data Type Conversion5/1(In1)
  t/1 -> outputs/1
  inputs/1 -> in15_repeat/1
  fitting_parameters/1 -> in4_repeat/1
  psi_pm/1 -> in7_repeat/1
  Lq/1 -> in5_repeat/1
  Ld/1 -> in6_repeat/1
  polepairs/1 -> in18_repeat/1
  R1/1 -> in9_repeat/1
  M_n0/1 -> in16_repeat/1
  mu/1 -> in0_repeat/1
  reciprocal_J/1 -> in13_repeat/1
  simulate_nonlinear/1 -> in2_repeat/1
  simulate_mechanical/1 -> in1_repeat/1
  reset_integrators/1 -> in10_repeat/1

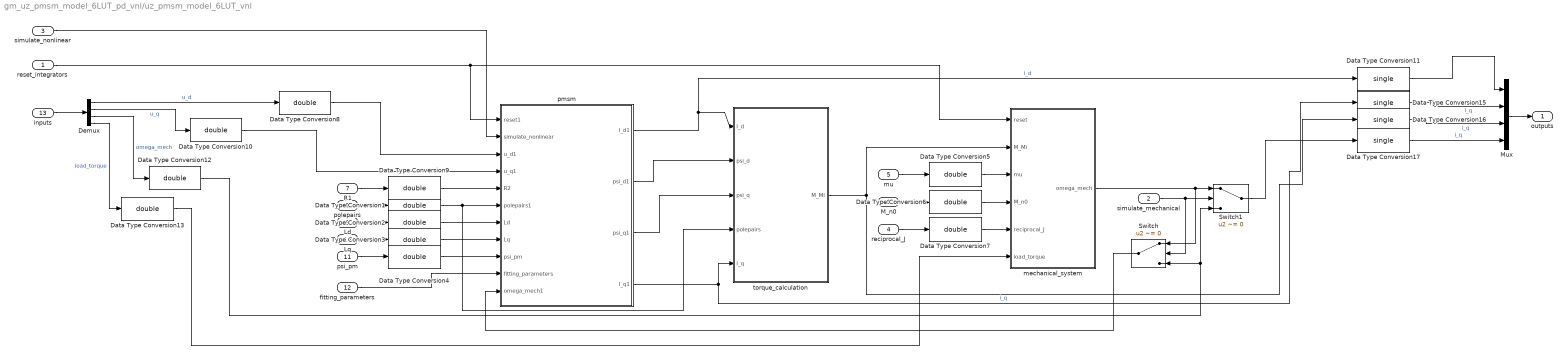
== system gm_uz_pmsm_model_6LUT_pd_vnl/uz_pmsm_model_6LUT_vnl ==
  reset_integrators : Inport
  simulate_mechanical : Inport  Port=2
  simulate_nonlinear : Inport  Port=3
  reciprocal_J : Inport  Port=4
  mu : Inport  Port=5
  M_n0 : Inport  Port=6
  R1 : Inport  Port=7
  polepairs : Inport  Port=8
  Ld : Inport  Port=9
  Lq : Inport  Port=10
  psi_pm : Inport  Port=11
  fitting_parameters : Inport  Port=12
  inputs : Inport  Port=13
  Data Type Conversion{1..10,12..13} (12 alike) : DataTypeConversion  OutDataTypeStr=double  RndMeth=Nearest  SaturateOnIntegerOverflow=off
  Data Type Conversion{11,15..17} (4 alike) : DataTypeConversion  OutDataTypeStr=single  RndMeth=Nearest  SaturateOnIntegerOverflow=off
  Demux : Demux
  Mux : Mux
  Switch : Switch  Criteria=u2 ~= 0  SaturateOnIntegerOverflow=off  InputSameDT=off
  Switch1 : Switch  Criteria=u2 ~= 0  SaturateOnIntegerOverflow=off  InputSameDT=off
  mechanical_system : Subsystem
  pmsm : Subsystem
  torque_calculation : Subsystem
  outputs : Outport
  wires:
  Data Type Conversion13/1 -> mechanical_system/6(load_torque)
  Data Type Conversion12/1 -> Switch/3, Switch1/3
  Data Type Conversion10/1 -> pmsm/4(u_q1)
  Data Type Conversion8/1 -> pmsm/3(u_d1)
  Data Type Conversion7/1 -> mechanical_system/5(reciprocal_J)
  Data Type Conversion6/1 -> mechanical_system/4(M_n0)
  Data Type Conversion5/1 -> mechanical_system/3(mu)
  Data Type Conversion4/1 -> pmsm/9(psi_pm)
  Data Type Conversion3/1 -> pmsm/8(Lq)
  Data Type Conversion2/1 -> pmsm/7(Ld)
  Data Type Conversion1/1 -> pmsm/6(polepairs1), torque_calculation/4(polepairs)
  Data Type Conversion9/1 -> pmsm/5(R2)
  fitting_parameters/1 -> pmsm/10(fitting_parameters)
  simulate_nonlinear/1 -> pmsm/2(simulate_nonlinear)
  Ld/1 -> Data Type Conversion2/1
  Lq/1 -> Data Type Conversion3/1
  psi_pm/1 -> Data Type Conversion4/1
  Mux/1 -> outputs/1
  inputs/1 -> Demux/1
  Data Type Conversion11/1 -> Mux/1
  Data Type Conversion15/1 -> Mux/2  "i_q"
  Data Type Conversion16/1 -> Mux/3  "i_q"
  Data Type Conversion17/1 -> Mux/4  "i_q"
  pmsm/1(I_d1) -> torque_calculation/1(I_d), Data Type Conversion11/1  "i_d"
  pmsm/4(I_q1) -> Data Type Conversion15/1, torque_calculation/5(I_q)  "i_q"
  mechanical_system/1(omega_mech) -> Switch1/1, Switch/1
  Demux/2 -> Data Type Conversion10/1  "u_q"
  M_n0/1 -> Data Type Conversion6/1
  torque_calculation/1(M_Mi) -> Data Type Conversion16/1, mechanical_system/2(M_Mi)
  reciprocal_J/1 -> Data Type Conversion7/1
  simulate_mechanical/1 -> Switch/2, Switch1/2
  mu/1 -> Data Type Conversion5/1
  Demux/1 -> Data Type Conversion8/1  "u_d"
  polepairs/1 -> Data Type Conversion1/1
  pmsm/3(psi_q1) -> torque_calculation/3(psi_q)
  R1/1 -> Data Type Conversion9/1
  Switch1/1 -> Data Type Conversion17/1
  Demux/4 -> Data Type Conversion13/1  "load_torque"
  pmsm/2(psi_d1) -> torque_calculation/2(psi_d)
  Switch/1 -> pmsm/11(omega_mech1)
  Demux/3 -> Data Type Conversion12/1  "omega_mech"
  reset_integrators/1 -> mechanical_system/1(reset), pmsm/1(reset1)

== system gm_uz_pmsm_model_6LUT_pd_vnl/Compare/Assert_outputs ==
  cosim : Inport
  dut : Inport  Port=2
  AssertEq : Assertion  StopWhenAssertionFail=off
  Compare To Zero : simulink/Logic and Bit Operations/Compare To Zero  relop===  OutDataTypeStr=boolean
  Constant1 : Constant  Value=0  OutDataTypeStr=Inherit: Inherit via back propagation  SampleTime=-1
  Counter : simulink/Sources/Counter Free-Running  NumBits=32  tsamp=-1
  IgnoreCycles : Constant  Value=2  OutDataTypeStr=Inherit: Inherit via back propagation  SampleTime=-1
  RelErrCheck : Subsystem
  Relational Operator : RelationalOperator  Operator=<  OutDataTypeStr=boolean  InputSameDT=off
  Switch : Switch  Criteria=u2 ~= 0  SaturateOnIntegerOverflow=off  InputSameDT=off
  Switch1 : Switch  Criteria=u2 ~= 0  SaturateOnIntegerOverflow=off  InputSameDT=off
  compare: outputs : Scope  NumInputPorts=3
  wires:
  IgnoreCycles/1 -> Relational Operator/2
  Counter/1 -> Relational Operator/1
  dut/1 -> Switch/3  "dut ref"
  cosim/1 -> Switch1/3  "cosim"
  Relational Operator/1 -> Switch1/2, Switch/2
  Constant1/1 -> Switch1/1, Switch/1
  Switch/1 -> compare: outputs/2, RelErrCheck/2(In2)
  Switch1/1 -> compare: outputs/1, RelErrCheck/1(In1)
  RelErrCheck/1(Out1) -> AssertEq/1, Compare To Zero/1  "err"
  Compare To Zero/1 -> compare: outputs/3

== system gm_uz_pmsm_model_6LUT_pd_vnl/Compare/CleanupScopes ==

== system gm_uz_pmsm_model_6LUT_pd_vnl/Compare/Enable ==

== system gm_uz_pmsm_model_6LUT_pd_vnl/Current_Controller/Entkopplung_flags ==
  u_d_static : Inport
  u_q_static : Inport  Port=2
  u_d_praed : Inport  Port=3
  u_q_praed : Inport  Port=4
  u_d_lin : Inport  Port=5
  u_q_lin : Inport  Port=6
  u_d_dyn : Inport  Port=7
  u_q_dyn : Inport  Port=8
  0 : Constant  Value=0
  Switch{1..8} (8 alike) : Switch  Criteria=u2 > Threshold  SaturateOnIntegerOverflow=off  InputSameDT=off
  entkopplung_dynamic : Constant  Value=entkopplung_dynamic
  entkopplung_linear : Constant  Value=entkopplung_linear
  entkopplung_preadiktion : Constant  Value=praediktion_entkopplung_nonlinear
  entkopplung_static : Constant  Value=entkopplung_static
  u_d_entk : Outport
  u_q_entk : Outport  Port=2
  wires:
  Switch3/1 -> u_d_entk/1
  Switch4/1 -> Switch2/3
  entkopplung_preadiktion/1 -> Switch2/2, Switch3/2
  Switch1/1 -> Switch3/3
  u_d_praed/1 -> Switch3/1
  Switch2/1 -> u_q_entk/1
  u_q_praed/1 -> Switch2/1
  entkopplung_static/1 -> Switch4/2, Switch1/2
  u_d_static/1 -> Switch1/1
  u_d_lin/1 -> Switch5/1
  Switch5/1 -> Switch1/3
  entkopplung_linear/1 -> Switch6/2, Switch5/2
  entkopplung_dynamic/1 -> Switch8/2, Switch7/2
  0/1 -> Switch8/3, Switch7/3
  Switch6/1 -> Switch4/3
  u_q_static/1 -> Switch4/1
  u_q_lin/1 -> Switch6/1
  u_d_dyn/1 -> Switch7/1
  Switch8/1 -> Switch6/3
  u_q_dyn/1 -> Switch8/1
  Switch7/1 -> Switch5/3

== system gm_uz_pmsm_model_6LUT_pd_vnl/Current_Controller/Entkopplungen ==
  u_q : Inport
  u_d : Inport  Port=2
  uq : Inport  Port=3
  ud : Inport  Port=4
  i_d : Inport  Port=5
  psi_d_LUT : Inport  Port=6
  psi_q_LUT : Inport  Port=7
  Ldq_LUT : Inport  Port=8
  Lqd_LUT : Inport  Port=9
  i_q : Inport  Port=10
  omega_m : Inport  Port=11
  Lineare_Entkopplung : Subsystem
  decoupling_praediktion : Subsystem
  dynamic_nonlinear_entkopplung1 : Subsystem
  static_nonlinear_entkopplung : Subsystem
  u_d_static : Outport
  u_q_static : Outport  Port=2
  u_d_prae : Outport  Port=3
  u_q_prae : Outport  Port=4
  u_d_lin : Outport  Port=5
  u_q_lin : Outport  Port=6
  u_d_dyn : Outport  Port=7
  u_q_dyn1 : Outport  Port=8
  wires:
  psi_d_LUT/1 -> static_nonlinear_entkopplung/1(psi_d), dynamic_nonlinear_entkopplung1/3(psi_d), decoupling_praediktion/9(psi_d)
  omega_m/1 -> dynamic_nonlinear_entkopplung1/7(omega_m), Lineare_Entkopplung/3(omega_m), static_nonlinear_entkopplung/3(omega_m), decoupling_praediktion/5(omega_m)
  psi_q_LUT/1 -> dynamic_nonlinear_entkopplung1/4(psi_q), decoupling_praediktion/8(psi_q), static_nonlinear_entkopplung/2(psi_q)
  u_q/1 -> decoupling_praediktion/4(u_q_1)
  i_d/1 -> dynamic_nonlinear_entkopplung1/1(i_d), Lineare_Entkopplung/1(i_d), decoupling_praediktion/1(i_d)
  i_q/1 -> dynamic_nonlinear_entkopplung1/2(i_q), Lineare_Entkopplung/2(i_q), decoupling_praediktion/3(i_q)
  ud/1 -> decoupling_praediktion/6(u_d_k)
  uq/1 -> decoupling_praediktion/7(u_q_k)
  u_d/1 -> decoupling_praediktion/2(u_d_1)
  static_nonlinear_entkopplung/1(u_d) -> u_d_static/1
  Lineare_Entkopplung/1(u_d) -> u_d_lin/1
  static_nonlinear_entkopplung/2(u_q) -> u_q_static/1
  decoupling_praediktion/1(u_d_entk) -> u_d_prae/1
  Lineare_Entkopplung/2(u_q) -> u_q_lin/1
  decoupling_praediktion/2(u_q_entk) -> u_q_prae/1
  dynamic_nonlinear_entkopplung1/1(u_d) -> u_d_dyn/1
  dynamic_nonlinear_entkopplung1/2(u_q) -> u_q_dyn1/1
  Ldq_LUT/1 -> dynamic_nonlinear_entkopplung1/5(Ldq_LUT)
  Lqd_LUT/1 -> dynamic_nonlinear_entkopplung1/6(Lqd_LUT)
